simulink library "libH7_6DOF"  (R2021b)
settings: Solver=VariableStepAuto  StartTime=0.0  StopTime=10.0  RelTol=1e-3
undefined symbols (not defined in the file or in its folder): pod
libraries: shared6dof x1, $bdroot x1
settings Model: Creator=Ferran  LastModifiedBy=Ferran

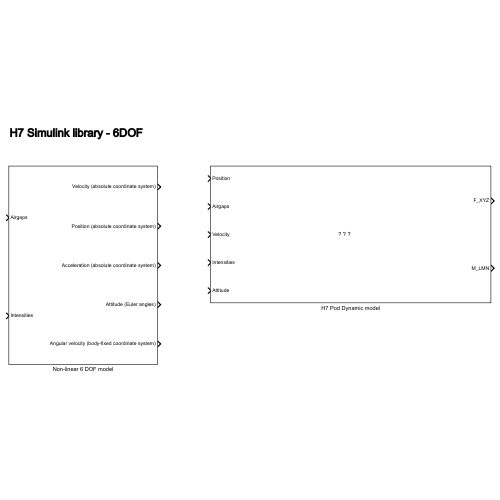
[thumbnail: Simulink's stored preview of the top-level diagram]
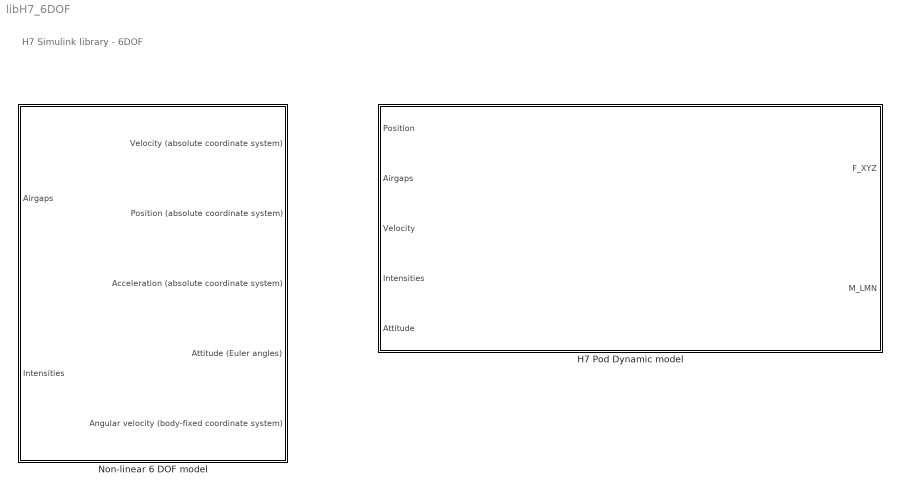
== system libH7_6DOF ==
  note: H7 Simulink library - 6DOF
  H7 Pod Dynamic model : Subsystem
      mask Display: image('FBD.png', [0.12 0.12 0.78 0.78]); % Use "Edit Image" on toolstrip to change.
  Non-linear 6 DOF model : Subsystem

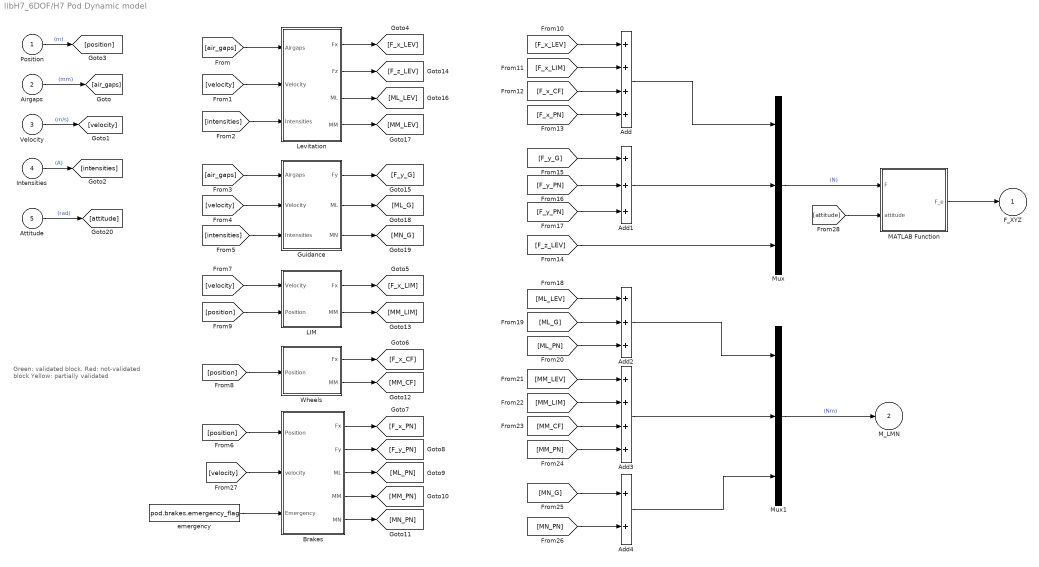
== system libH7_6DOF/H7 Pod Dynamic model ==
  note: Green: validated block.
      | Red: not-validated block
      | Yellow: partially validated
  Position : Inport
  Airgaps : Inport  Port=2
  Velocity : Inport  Port=3
  Intensities : Inport  Port=4
  Attitude : Inport  Port=5
  Add : Sum  Inputs=++++
  Add1 : Sum  Inputs=+++
  Add2 : Sum  Inputs=+++
  Add3 : Sum  Inputs=++++
  Add4 : Sum
  Brakes : Subsystem
  Guidance : Subsystem
  LIM : Subsystem
  Levitation : Subsystem
  MATLAB Function : MATLAB Function  TreatAsAtomicUnit=on
  Mux : Mux  Inputs=3
  Mux1 : Mux  Inputs=3
  Wheels : Subsystem
  emergency : Constant  Value=pod.brakes.emergency_flag
  F_XYZ : Outport
  M_LMN : Outport  Port=2
  wires:
  Airgaps/1 -> [air_gaps]  "(mm)"
  Velocity/1 -> [velocity]  "(m/s)"
  Intensities/1 -> [intensities]  "(A)"
  Mux/1 -> MATLAB Function/1(F)  "(N)"
  Mux1/1 -> M_LMN/1  "(Nm)"
  [air_gaps] -> Levitation/1(Airgaps)
  [velocity] -> Levitation/2(Velocity)
  [intensities] -> Levitation/3(Intensities)
  [velocity] -> Guidance/2(Velocity)
  [intensities] -> Guidance/3(Intensities)
  [air_gaps] -> Guidance/1(Airgaps)
  [velocity] -> LIM/1(Velocity)
  Position/1 -> [position]  "(m)"
  [position] -> Brakes/1(Position)
  emergency/1 -> Brakes/3(Emergency)
  [position] -> Wheels/1(Position)
  [position] -> LIM/2(Position)
  Levitation/1(Fx) -> [F_x_LEV]
  LIM/1(Fx) -> [F_x_LIM]
  Wheels/1(Fx) -> [F_x_CF]
  Brakes/1(Fx) -> [F_x_PN]
  Brakes/2(Fy) -> [F_y_PN]
  Brakes/3(ML) -> [ML_PN]
  Brakes/4(MM) -> [MM_PN]
  Brakes/5(MN) -> [MN_PN]
  Wheels/2(MM) -> [MM_CF]
  LIM/2(MM) -> [MM_LIM]
  Levitation/2(Fz) -> [F_z_LEV]
  Guidance/1(Fy) -> [F_y_G]
  Levitation/3(ML) -> [ML_LEV]
  Levitation/4(MM) -> [MM_LEV]
  Guidance/2(ML) -> [ML_G]
  Guidance/3(MN) -> [MN_G]
  Add/1 -> Mux/1
  [F_x_LEV] -> Add/1
  [F_x_LIM] -> Add/2
  [F_x_CF] -> Add/3
  [F_x_PN] -> Add/4
  [F_z_LEV] -> Mux/3
  [F_y_G] -> Add1/1
  [F_y_PN] -> Add1/2
  [F_y_PN] -> Add1/3
  Add1/1 -> Mux/2
  [ML_LEV] -> Add2/1
  Add2/1 -> Mux1/1
  [ML_G] -> Add2/2
  [ML_PN] -> Add2/3
  [MM_LEV] -> Add3/1
  [MM_PN] -> Add3/4
  Add3/1 -> Mux1/2
  [MM_LIM] -> Add3/2
  [MM_CF] -> Add3/3
  [MN_PN] -> Add4/2
  [MN_G] -> Add4/1
  Add4/1 -> Mux1/3
  [velocity] -> Brakes/2(velocity)
  Attitude/1 -> [attitude]  "(rad)"
  [attitude] -> MATLAB Function/2(attitude)
  MATLAB Function/1(F_e) -> F_XYZ/1

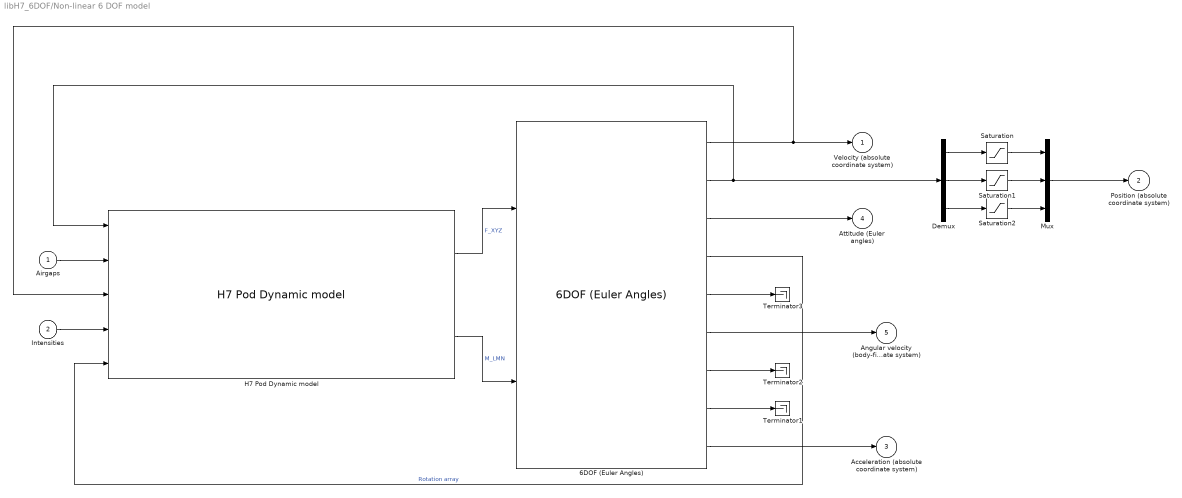
== system libH7_6DOF/Non-linear 6 DOF model ==
  Airgaps : Inport
  Intensities : Inport  Port=2
  6DOF (Euler Angles) : shared6dof/6DOF (Euler Angles)  units=Metric (MKS)  mtype=Fixed  rep=Euler Angles  xme_0=initial_conds.x_0  Vm_0=initial_conds.v_0  eul_0=initial_conds.ang_0  pm_0=initial_conds.w_0  mass_0=pod.mass.mass  mass_e=0.5  mass_f=2.0  inertia=pod.mass.inertia  inertia_e=eye(3)  inertia_f=2*eye(3)  k_quat=1.0  vre_flag=on  abi_flag=on  aMode=0  xme_statename=''  Vm_statename=''  eul_statename=''  quat_statename=''  pm_statename=''  mass_statename=''
      link override Abi: Port=9
      settings: SourceProductBaseCode=AE,PW,DR,MT,UV,VE
  Demux : Demux  Outputs=3
  H7 Pod Dynamic model : $bdroot/H7 Pod Dynamic model  SystemSampleTime=-1  VariantActivationTime=update diagram  Latency=0  AutoFrameSizeCalculation=off
  Mux : Mux  Inputs=3
  Saturation : Saturate  UpperLimit=20  LowerLimit=0
  Saturation1 : Saturate  UpperLimit=0.002  LowerLimit=-0.002
  Saturation2 : Saturate  UpperLimit=0  LowerLimit=-0.011
  Terminator1 : Terminator
  Terminator2 : Terminator
  Terminator3 : Terminator
  Velocity (absolute coordinate system) : Outport
  Position (absolute coordinate system) : Outport  Port=2
  Acceleration (absolute coordinate system) : Outport  Port=3
  Attitude (Euler angles) : Outport  Port=4
  Angular velocity (body-fixed coordinate system) : Outport  Port=5
  wires:
  6DOF (Euler Angles)/2 -> Demux/1, H7 Pod Dynamic model/1
  6DOF (Euler Angles)/1 -> Velocity (absolute coordinate system)/1, H7 Pod Dynamic model/3
  Intensities/1 -> H7 Pod Dynamic model/4
  6DOF (Euler Angles)/4 -> H7 Pod Dynamic model/5  "Rotation array"
  H7 Pod Dynamic model/1 -> 6DOF (Euler Angles)/1  "F_XYZ"
  H7 Pod Dynamic model/2 -> 6DOF (Euler Angles)/2  "M_LMN"
  6DOF (Euler Angles)/8 -> Terminator1/1
  6DOF (Euler Angles)/6 -> Angular velocity (body-fixed coordinate system)/1
  6DOF (Euler Angles)/9 -> Acceleration (absolute coordinate system)/1
  6DOF (Euler Angles)/3 -> Attitude (Euler angles)/1
  6DOF (Euler Angles)/5 -> Terminator3/1
  6DOF (Euler Angles)/7 -> Terminator2/1
  Airgaps/1 -> H7 Pod Dynamic model/2
  Demux/1 -> Saturation/1
  Demux/2 -> Saturation1/1
  Demux/3 -> Saturation2/1
  Saturation/1 -> Mux/1
  Saturation1/1 -> Mux/2
  Saturation2/1 -> Mux/3
  Mux/1 -> Position (absolute coordinate system)/1

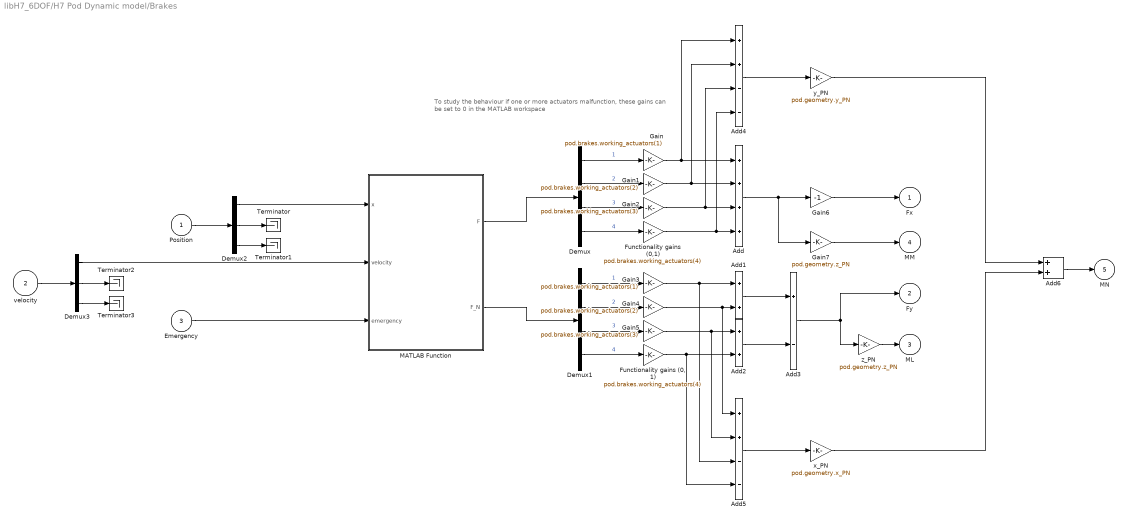
== system libH7_6DOF/H7 Pod Dynamic model/Brakes ==
  note: To study the behaviour if one or more actuators malfunction,
      | these gains can be set to 0 in the MATLAB workspace
  Position : Inport
  velocity : Inport  Port=2
  Emergency : Inport  Port=3
  Add : Sum  Inputs=++++
  Add1 : Sum
  Add2 : Sum
  Add3 : Sum  Inputs=+-
  Add4 : Sum  Inputs=++--
  Add5 : Sum  Inputs=++--
  Add6 : Sum
  Demux : Demux
  Demux1 : Demux
  Demux2 : Demux  Outputs=3
  Demux3 : Demux  Outputs=3
  "Functionality gains (0, 1)" : Gain  Gain=pod.brakes.working_actuators(4)
  Functionality gains (0,1) : Gain  Gain=pod.brakes.working_actuators(4)
  Gain : Gain  Gain=pod.brakes.working_actuators(1)
  Gain1 : Gain  Gain=pod.brakes.working_actuators(2)
  Gain2 : Gain  Gain=pod.brakes.working_actuators(3)
  Gain3 : Gain  Gain=pod.brakes.working_actuators(1)
  Gain4 : Gain  Gain=pod.brakes.working_actuators(2)
  Gain5 : Gain  Gain=pod.brakes.working_actuators(3)
  Gain6 : Gain  Gain=-1
  Gain7 : Gain  Gain=pod.geometry.z_PN
  MATLAB Function : MATLAB Function  TreatAsAtomicUnit=on
  Terminator{,1..3} (4 alike) : Terminator
  x_PN : Gain  Gain=pod.geometry.x_PN
  y_PN : Gain  Gain=pod.geometry.y_PN
  z_PN : Gain  Gain=pod.geometry.z_PN
  Fx : Outport
  Fy : Outport  Port=2
  ML : Outport  Port=3
  MM : Outport  Port=4
  MN : Outport  Port=5
  wires:
  Emergency/1 -> MATLAB Function/3(emergency)
  MATLAB Function/1(F) -> Demux/1
  Demux/1 -> Gain/1  "1"
  Demux/2 -> Gain1/1  "2"
  Demux/3 -> Gain2/1  "3"
  Demux/4 -> Functionality gains (0,1)/1  "4"
  Demux1/4 -> "Functionality gains (0, 1)"/1  "4"
  Demux1/3 -> Gain5/1  "3"
  Demux1/1 -> Gain3/1  "1"
  Demux1/2 -> Gain4/1  "2"
  MATLAB Function/2(F_N) -> Demux1/1
  Functionality gains (0,1)/1 -> Add4/4, Add/4
  Gain2/1 -> Add4/3, Add/3
  Gain1/1 -> Add4/2, Add/2
  Gain/1 -> Add4/1, Add/1
  Add/1 -> Gain7/1, Gain6/1
  Gain6/1 -> Fx/1
  Gain4/1 -> Add5/1, Add1/2
  Gain3/1 -> Add1/1, Add5/3
  Gain5/1 -> Add5/2, Add2/1
  "Functionality gains (0, 1)"/1 -> Add2/2, Add5/4
  Add1/1 -> Add3/1
  Add2/1 -> Add3/2
  Add3/1 -> z_PN/1, Fy/1
  z_PN/1 -> ML/1
  Gain7/1 -> MM/1
  Add4/1 -> y_PN/1
  Demux2/3 -> Terminator1/1
  Position/1 -> Demux2/1
  Demux2/1 -> MATLAB Function/1(x)
  Demux2/2 -> Terminator/1
  velocity/1 -> Demux3/1
  Demux3/2 -> Terminator2/1
  Demux3/3 -> Terminator3/1
  Demux3/1 -> MATLAB Function/2(velocity)
  Add5/1 -> x_PN/1
  Add6/1 -> MN/1
  y_PN/1 -> Add6/1
  x_PN/1 -> Add6/2

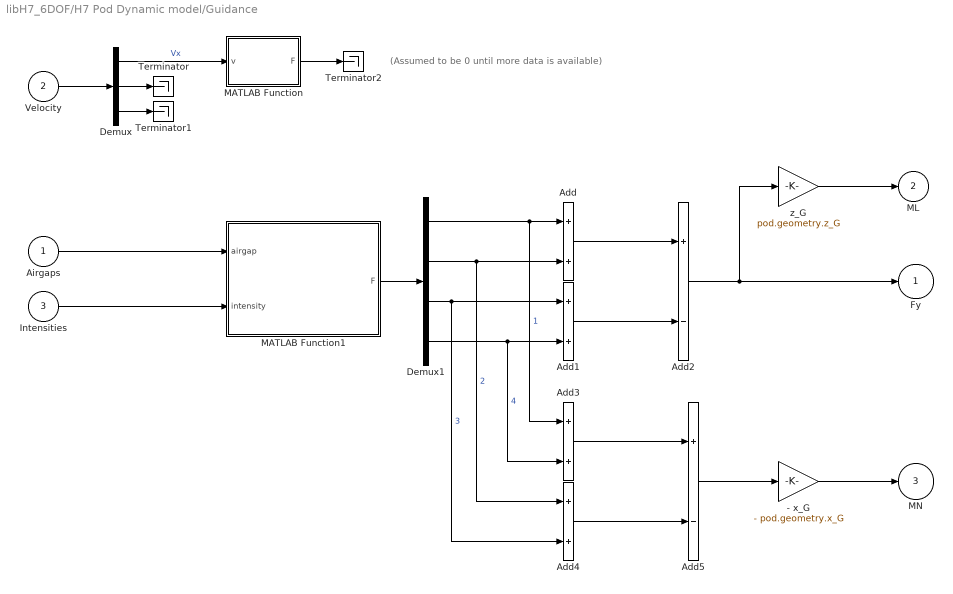
== system libH7_6DOF/H7 Pod Dynamic model/Guidance ==
  note: (Assumed to be 0 until more data is available)
  Airgaps : Inport
  Velocity : Inport  Port=2
  Intensities : Inport  Port=3
  - x_G : Gain  Gain=- pod.geometry.x_G
  Add{,1,3..4} (4 alike) : Sum
  Add2 : Sum  Inputs=+-
  Add5 : Sum  Inputs=+-
  Demux : Demux  Outputs=3
  Demux1 : Demux
  MATLAB Function : MATLAB Function  TreatAsAtomicUnit=on
  MATLAB Function1 : MATLAB Function  TreatAsAtomicUnit=on
  Terminator : Terminator
  Terminator1 : Terminator
  Terminator2 : Terminator
  z_G : Gain  Gain=pod.geometry.z_G
  Fy : Outport
  ML : Outport  Port=2
  MN : Outport  Port=3
  wires:
  Demux/1 -> MATLAB Function/1(v)  "Vx"
  Velocity/1 -> Demux/1
  Demux/2 -> Terminator/1
  Demux/3 -> Terminator1/1
  MATLAB Function/1(F) -> Terminator2/1
  MATLAB Function1/1(F) -> Demux1/1
  Intensities/1 -> MATLAB Function1/2(intensity)
  Airgaps/1 -> MATLAB Function1/1(airgap)
  Demux1/1 -> Add3/1, Add/1  "1"
  Demux1/2 -> Add4/1, Add/2  "2"
  Demux1/3 -> Add4/2, Add1/1  "3"
  Demux1/4 -> Add3/2, Add1/2  "4"
  Add1/1 -> Add2/2
  Add/1 -> Add2/1
  Add2/1 -> z_G/1, Fy/1
  z_G/1 -> ML/1
  Add3/1 -> Add5/1
  Add4/1 -> Add5/2
  Add5/1 -> - x_G/1
  - x_G/1 -> MN/1

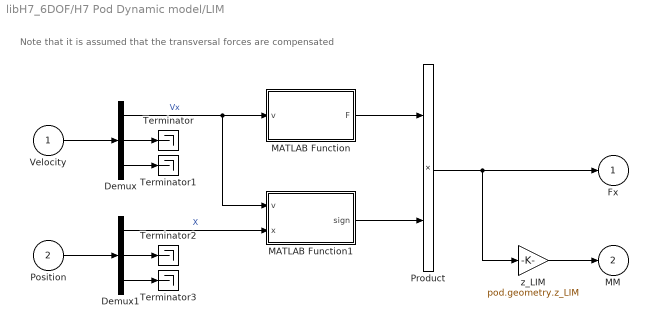
== system libH7_6DOF/H7 Pod Dynamic model/LIM ==
  note: Note that it is assumed that the transversal forces are compensated
  Velocity : Inport
  Position : Inport  Port=2
  Demux : Demux  Outputs=3
  Demux1 : Demux  Outputs=3
  MATLAB Function : MATLAB Function  TreatAsAtomicUnit=on
  MATLAB Function1 : MATLAB Function  TreatAsAtomicUnit=on
  Product : Product
  Terminator{,1..3} (4 alike) : Terminator
  z_LIM : Gain  Gain=pod.geometry.z_LIM
  Fx : Outport
  MM : Outport  Port=2
  wires:
  Velocity/1 -> Demux/1
  Demux/2 -> Terminator/1
  Demux/3 -> Terminator1/1
  Demux/1 -> MATLAB Function1/1(v), MATLAB Function/1(v)  "Vx"
  Position/1 -> Demux1/1
  Demux1/3 -> Terminator3/1
  Demux1/2 -> Terminator2/1
  Demux1/1 -> MATLAB Function1/2(x)  "X"
  MATLAB Function1/1(sign) -> Product/2
  MATLAB Function/1(F) -> Product/1
  Product/1 -> z_LIM/1, Fx/1
  z_LIM/1 -> MM/1

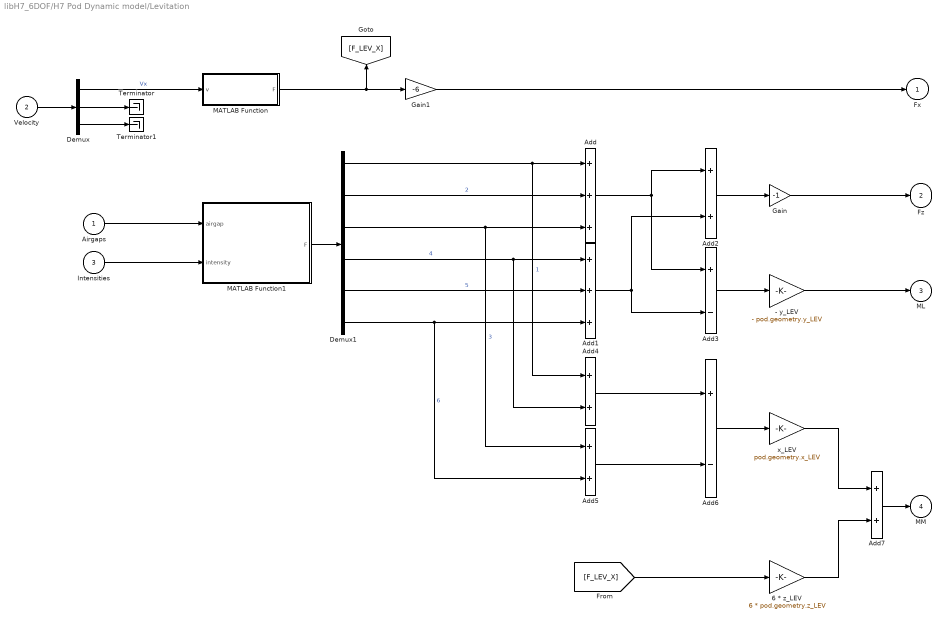
== system libH7_6DOF/H7 Pod Dynamic model/Levitation ==
  Airgaps : Inport
  Velocity : Inport  Port=2
  Intensities : Inport  Port=3
  - y_LEV : Gain  Gain=- pod.geometry.y_LEV
  6 * z_LEV : Gain  Gain=6 * pod.geometry.z_LEV
  Add : Sum  Inputs=+++
  Add1 : Sum  Inputs=+++
  Add{2,4..5,7} (4 alike) : Sum
  Add3 : Sum  Inputs=+-
  Add6 : Sum  Inputs=+-
  Demux : Demux  Outputs=3
  Demux1 : Demux  Outputs=6
  Gain : Gain  Gain=-1
  Gain1 : Gain  Gain=-6
  MATLAB Function : MATLAB Function  TreatAsAtomicUnit=on
  MATLAB Function1 : MATLAB Function  TreatAsAtomicUnit=on
  Terminator : Terminator
  Terminator1 : Terminator
  x_LEV : Gain  Gain=pod.geometry.x_LEV
  Fx : Outport
  Fz : Outport  Port=2
  ML : Outport  Port=3
  MM : Outport  Port=4
  wires:
  Demux/2 -> Terminator/1
  Demux/3 -> Terminator1/1
  Velocity/1 -> Demux/1
  Demux/1 -> MATLAB Function/1(v)  "Vx"
  Airgaps/1 -> MATLAB Function1/1(airgap)
  Intensities/1 -> MATLAB Function1/2(intensity)
  MATLAB Function1/1(F) -> Demux1/1
  Gain/1 -> Fz/1
  Demux1/1 -> Add4/1, Add/1  "1"
  Demux1/2 -> Add/2  "2"
  Demux1/3 -> Add5/1, Add/3  "3"
  Demux1/4 -> Add4/2, Add1/1  "4"
  Demux1/5 -> Add1/2  "5"
  Demux1/6 -> Add5/2, Add1/3  "6"
  Add/1 -> Add2/1, Add3/1
  Add1/1 -> Add2/2, Add3/2
  Add2/1 -> Gain/1
  Add3/1 -> - y_LEV/1
  - y_LEV/1 -> ML/1
  Gain1/1 -> Fx/1
  [F_LEV_X] -> 6 * z_LEV/1
  Add4/1 -> Add6/1
  Add5/1 -> Add6/2
  Add6/1 -> x_LEV/1
  Add7/1 -> MM/1
  x_LEV/1 -> Add7/1
  6 * z_LEV/1 -> Add7/2
  MATLAB Function/1(F) -> [F_LEV_X], Gain1/1

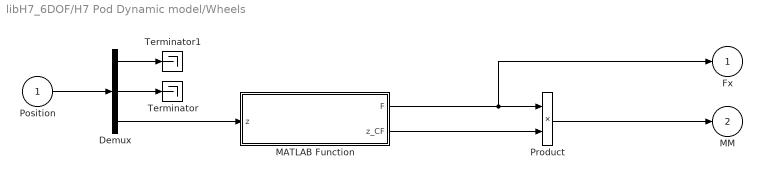
== system libH7_6DOF/H7 Pod Dynamic model/Wheels ==
  Position : Inport
  Demux : Demux  Outputs=3
  MATLAB Function : MATLAB Function  TreatAsAtomicUnit=on
  Product : Product
  Terminator : Terminator
  Terminator1 : Terminator
  Fx : Outport
  MM : Outport  Port=2
  wires:
  Position/1 -> Demux/1
  Demux/2 -> Terminator/1
  Demux/3 -> MATLAB Function/1(z)
  MATLAB Function/1(F) -> Fx/1, Product/1
  Demux/1 -> Terminator1/1
  MATLAB Function/2(z_CF) -> Product/2
  Product/1 -> MM/1

== matlab function libH7_6DOF/H7 Pod Dynamic model/Levitation/MATLAB Function ==
  data: v input; F output; pod parameter
function F = HEMSdrag(v, pod)
% Computes the drag force (N) of one HEMS unit as a function of the 
% velocity (m/s)
% ═════════════════════════════════════════════════════════════════════════
% Last updated: 15.12.2021
% ═════════════════════════════════════════════════════════════════════════

F = pod.levitation.drag_1_unit.poly.p3*v^3 + ...
    pod.levitation.drag_1_unit.poly.p2*v^2 + ...
    pod.levitation.drag_1_unit.poly.p1*v   + ...
    pod.levitation.drag_1_unit.poly.p0;

== matlab function libH7_6DOF/H7 Pod Dynamic model/MATLAB Function ==
  data: F input; F_e output; attitude input; pod parameter
function F_e = BF2E(F, attitude, pod)
% Computes the total force in absoute axis
% ═════════════════════════════════════════════════════════════════════════
% Last updated: 27.12.2021
% ═════════════════════════════════════════════════════════════════════════
F     = reshape(F, [3 1]);


F_e = attitude * F + pod.mass.mass * [0 0 9.81]';

== matlab function libH7_6DOF/H7 Pod Dynamic model/Levitation/MATLAB Function1 ==
  data: airgap input; F output; intensity input; pod parameter
function F = HEMSlev(airgap, intensity, pod)
% Computes the levitation force (N) of all the HEMS units as a function of 
% their air gaps (mm) and intensities (A)
% ═════════════════════════════════════════════════════════════════════════
% Last updated: 15.12.2021
% ════════════════════════════════════════════════════════════════════════

x   = airgap(1:6);
y   = intensity(1:6);

F = pod.levitation.poly_1_unit.p00 + ...
    pod.levitation.poly_1_unit.p10.*x + ...
    pod.levitation.poly_1_unit.p01.*y + ...
    pod.levitation.poly_1_unit.p20.*x.^2 + ...
    pod.levitation.poly_1_unit.p11.*x.*y + ...
    pod.levitation.poly_1_unit.p02.*y.^2 + ...
    pod.levitation.poly_1_unit.p21.*x.^2.*y + ...
    pod.levitation.poly_1_unit.p12.*x.*y.^2 + ...
    pod.levitation.poly_1_unit.p03.*y.^3;

== matlab function libH7_6DOF/H7 Pod Dynamic model/Guidance/MATLAB Function ==
  data: v input; F output
function F = EMSdrag(v)
% Computes the drag force (N) of one EMS units as a function of 
% its velocity (m/s)
% ═════════════════════════════════════════════════════════════════════════
% Last updated: 15.12.2021
% ════════════════════════════════════════════════════════════════════════

F = 0;

== matlab function libH7_6DOF/H7 Pod Dynamic model/Guidance/MATLAB Function1 ==
  data: airgap input; F output; intensity input; pod parameter
function F = EMSlev(airgap, intensity, pod)
% Computes the levitation force (N) of all the EMS units as a function of 
% their air gaps (mm) and intensities (A)
% ═════════════════════════════════════════════════════════════════════════
% Last updated: 15.12.2021
% ════════════════════════════════════════════════════════════════════════

x   = airgap(7:10);
y   = intensity(7:10);

F = pod.guiding.poly.p00 + ...
    pod.guiding.poly.p10.*x + ...
    pod.guiding.poly.p01.*y + ...
    pod.guiding.poly.p20.*x.^2 + ...
    pod.guiding.poly.p11.*x.*y + ...
    pod.guiding.poly.p02.*y.^2 + ...
    pod.guiding.poly.p21.*x.^2.*y + ...
    pod.guiding.poly.p12.*x.*y.^2 + ...
    pod.guiding.poly.p03.*y.^3;

== matlab function libH7_6DOF/H7 Pod Dynamic model/LIM/MATLAB Function ==
  data: v input; F output; pod parameter
function F = LIMtraction(v, pod)
% Computes the traction force (N) of the LIM as a function of 
% the absolute velocity of the prototype (m/s)
% ═════════════════════════════════════════════════════════════════════════
% Last updated: 20.12.2021
% ═════════════════════════════════════════════════════════════════════════

F = pod.propulsion.poly.p3*v^3 + ...
    pod.propulsion.poly.p2*v^2 + ...
    pod.propulsion.poly.p1*v   + ...
    pod.propulsion.poly.p0;

== matlab function libH7_6DOF/H7 Pod Dynamic model/LIM/MATLAB Function1 ==
  data: v input; x input; sign output; pod parameter
function sign = LIMdirection(v, x, pod)
% Decides if the LIM force is being applied to accelerate or to brake 
% by comparing the position of the pod with a predefined treshold
% ═════════════════════════════════════════════════════════════════════════
% Last updated: 20.12.2021
% ═════════════════════════════════════════════════════════════════════════

if x >= pod.brakes.d && v > 0    
    sign = -1;
elseif x >= pod.brakes.d && v <= 0
    sign = 0;
else
    sign = 1;
end

== matlab function libH7_6DOF/H7 Pod Dynamic model/Wheels/MATLAB Function ==
  data: z input; F output; pod parameter; z_CF output
function [F, z_CF] = rollingFriction(z, pod)
% Computes the rolling resistance force (N) of the wheels. It distinguishes
% 3 cases: 
%   (1) z = 0. Pod touching the ground
%   (2) z = z_max. Pod touching the ceiling. It is assumed no current
%   applied to the HEMS. 
%   (3) Otherwise. Pod levitating. 
% ═════════════════════════════════════════════════════════════════════════
% Last updated: 26.12.2021
% ═════════════════════════════════════════════════════════════════════════

% F_LEV worst case scenario computation
x   = 12; % [mm]
y   = 0;  % [A]

F_LEV = pod.levitation.poly_1_unit.p00 + ...
        pod.levitation.poly_1_unit.p10.*x + ...
        pod.levitation.poly_1_unit.p01.*y + ...
        pod.levitation.poly_1_unit.p20.*x.^2 + ...
        pod.levitation.poly_1_unit.p11.*x.*y + ...
        pod.levitation.poly_1_unit.p02.*y.^2 + ...
        pod.levitation.poly_1_unit.p21.*x.^2.*y + ...
        pod.levitation.poly_1_unit.p12.*x.*y.^2 + ...
        pod.levitation.poly_1_unit.p03.*y.^3;

% Main algorithm
if z == 0
    F_N   = pod.mass.mass * 9.81;
    z_CF  = - pod.geometry.z_CF;
elseif z == pod.general.z_range
    F_N   = 6 * F_LEV - pod.mass.mass * 9.81;
    z_CF  = pod.geometry.z_CF;
else
    F_N   = 0;
    z_CF  = 0;
end

F = pod.wheels.number * pod.wheels.roll_coef * F_N;

== matlab function libH7_6DOF/H7 Pod Dynamic model/Brakes/MATLAB Function ==
  data: x input; velocity input; F output; emergency input; F_N output; pod parameter
function [F, F_N] = brakes_activation(x, velocity, emergency, pod)
% Computes the braking force of the pneumatic actuators if and only if 
%     (1) The emergency flag has been raised
%     (2) The pod is above the acceleration phase distance
% ═════════════════════════════════════════════════════════════════════════
% Last updated: 20.12.2021
% ═════════════════════════════════════════════════════════════════════════

if (emergency == 1 && x >= pod.brakes.d && velocity >= 0)
    F       = pod.brakes.force * ones(pod.brakes.n,1);
    F_N     = pod.brakes.normal_force * ones(pod.brakes.n,1);
else
    F       = zeros(pod.brakes.n,1);
    F_N     = zeros(pod.brakes.n,1);
end
